simulink model "sim12xx1"  (Simulink 4.00)
settings: Solver=ode45  SolverMode=SingleTasking  StartTime=0.0  StopTime=2  MaxStep=.010  RelTol=1e-3  AbsTol=1e-3
values from neighbouring files (symbols this model uses):
  k = length(a1)    [Chp2ex6.m]    (also in Chp6fig3.m = 3; Chp6fig4.m = 3; Chp6fig5.m = 3; Decouple.m = 2)
settings Model: LastModifiedBy=saadat  SaveTime=off  SaveOutput=off  LimitDataPoints=off  RTWTemplateMakefile=grt_vc.tmf  ExtModeTrigMode=oneshot  ExtModeArmWhenConnect=off

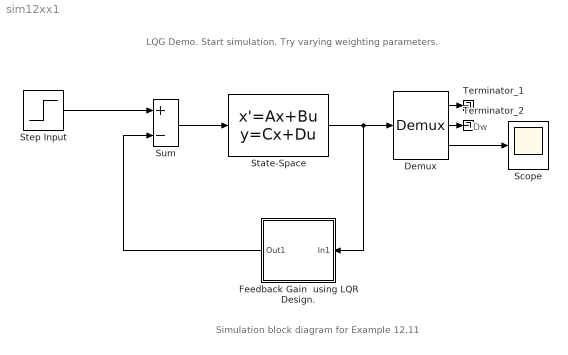
== system sim12xx1 ==
  note: Simulation block diagram for Example 12.11
  note: Dw
  note: LQG Demo. Start simulation.
      | Try varying weighting parameters.
  Demux : Demux  Outputs=3  BusSelectionMode=off
  Feedback Gain  using LQR Design. : Subsystem  Orientation=left  mask(Regulator){@1=[-5   0   -100;  2   -2    0;   0    0.1   -0.08], @2=[0;   0;    -0.1], @3=eye(3), @4=zeros(3,1), @5=[20, 0  0;  0  10   0;  0   0   5], @6=eye(1,1)*.15}
      mask prompts: @1 "Plant A matrix:"; @2 "Plant B matrix:"; @3 "Plant C matrix:"; @4 "Plant D matrix:"; @5 "Output weighting, y'Qy:"; @6 "Input weighting, u'Ru:"
      mask help:
      | Linear quadratic regulator.
      | (Requires Control Toolbox)
      mask init:
      | [k]=lqry(@1,@2,@3,@4,@5,@6);
      settings: RTWFcnNameOpts=Auto  RTWFileNameOpts=Auto
      mask Help: Implements a linear state quadratic regulator. Mask and unmask this block to see how it works.
      mask Display: disp('K')
  Scope : Scope
      settings: TickLabels=on  TimeRange=2  YMin=-0.0012  YMax=0  SaveToWorkspace=off  SaveName=ScopeData  DataFormat=Array  LimitDataPoints=on  MaxDataPoints=5000
  State-Space : StateSpace  A="[-5  0  -100;  2  -2  0;  0  0.1  -0.08]"  B="[0;   0 ;  -0.1]"  C=eye(3)  D=zeros(3, 1)  X0=0  AbsoluteTolerance=auto  Realization=auto
  Step Input : Step  Time=0  Before=0  After=.2  SampleTime=0
  Sum : Sum  Inputs=+-  SaturateOnIntegerOverflow=on
  Terminator_1 : Terminator
  Terminator_2 : Terminator
  wires:
  Sum/1 -> State-Space/1
  Step Input/1 -> Sum/1
  Demux/3 -> Scope/1
  State-Space/1 -> Demux/1, Feedback Gain  using LQR Design./1(In1)
  Feedback Gain  using LQR Design./1(Out1) -> Sum/2
  Demux/1 -> Terminator_1/1
  Demux/2 -> Terminator_2/1

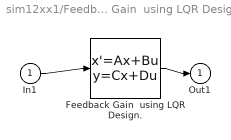
== system sim12xx1/Feedback Gain  using LQR Design. ==
  In1 : Inport  Port=1  LatchInput=off
  Feedback Gain  using LQR Design. : StateSpace  A=[]  B=[]  C=[]  D=k  X0=0  AbsoluteTolerance=auto  Realization=auto
  Out1 : Outport  Port=1
  wires:
  In1/1 -> Feedback Gain  using LQR Design./1
  Feedback Gain  using LQR Design./1 -> Out1/1
